simulink model "mosfetbuck_fre"  (R2014a)
settings: Solver=ode23tb  StartTime=0.0  StopTime=0.01  FixedStep=1e-08  RelTol=1e-4
PreLoadFcn:
  | %% Set up model sampling rate
  | Ts = 1e-7;
PostLoadFcn:
  | %% Compute the analytic transfer function for comparison purposes
  | % Load model quiecent operating conditions
  | Vin = str2double(get_param('mosfetbuck_fre/DC','Amplitude'));  % input voltage
  | Dq = str2double(get_param('mosfetbuck_fre/Dq','Value'));       % quiecent duty cycle
  | 
  | % Load model parameters
  | L = str2double(get_param('mosfetbuck_fre/L','Inductance'));    % Henrys
  | C = str2double(get_param('mosfetbuck_fre/C','Capacitance'));   % Farads
  | R = str2double(get_param('mosfetbuck_fre/Load','Resistance')); % Ohms
  | 
  | % Compute transfer function
  | GDnum = 1;
  | GDden = [L*C, L/R,1];
  | GD0 = Vin;
  | 
  | GDbuck = GD0*tf(GDnum,GDden);
InitFcn:
  | %% Set up model sampling rate
  | Ts = 1e-7;
libraries: powerlib x10, powerlib_meascontrol x1
settings Model: Creator=cosorio  LastModifiedBy=cosorio
settings DataIOCC: LimitDataPoints=off  SaveOutput=off  SignalLogging=off  SaveTime=off
settings OptimizationCC: ExpressionDepthLimit=2147483647
settings DebuggingCC: UnderspecifiedInitializationDetection=Classic  SolverPrmCheckMsg=none  FcnCallInpInsideContextMsg=UseLocalSettings  StateNameClashWarn=warning
settings GRTTargetCC: CombineOutputUpdateFcns=off  GRTInterface=on

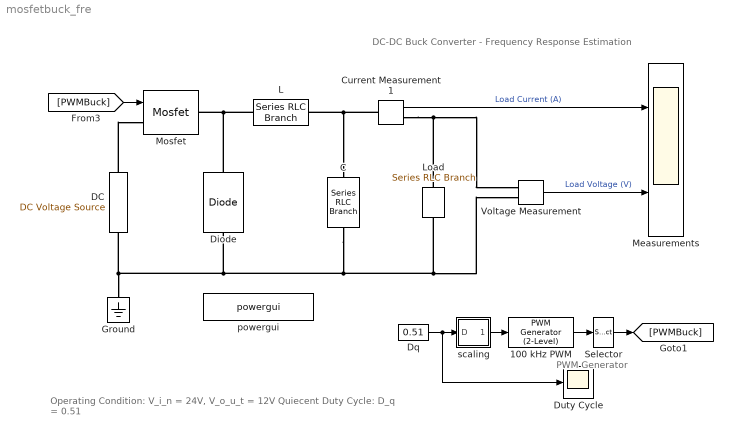
== system mosfetbuck_fre ==
  note: DC-DC Buck Converter - Frequency Response Estimation
  note: Operating Condition: V_i_n = 24V, V_o_u_t = 12V
      | Quiecent Duty Cycle: D_q = 0.51
  note: PWM Generator
  100 kHz PWM : powerlib_meascontrol/Pulse & Signal Generators/PWM Generator (2-Level)  ModulatorType=Single-phase half-bridge (2 pulses)  ModulatorMode=Unsynchronized  nF=27  Fc=1e5  ModulatingSignals=off  m=0.8  Freq=60  Phase=0  Ts=Ts
  C : powerlib/Elements/Series RLC Branch  LConnTagsString=__new0  RConnTagsString=__new0  BranchType=RC  Resistance=0.005  Inductance=30e-6  SetiL0=off  InitialCurrent=0  Capacitance=120e-6  Setx0=off  InitialVoltage=0  Measurements=None
  Current Measurement1 : powerlib/Measurements/Current Measurement  PhasorSimulation=off  OutputType=Complex  PSBequivalent=0
  DC : powerlib/Electrical Sources/DC Voltage Source  Amplitude=24  Measurements=None
  Diode : powerlib/Power Electronics/Diode  Ron=0.01  Lon=0  Vf=0.7  IC=0  UseSnubber=off  Rs=1e5  Cs=250e-9  Measurements=off
  Dq : Constant  Value=0.51  SampleTime=Ts
  Duty Cycle : Scope
      settings: YMin=0  YMax=1  SaveName=DutyCycle  Decimation=10
  Ground : powerlib/Elements/Ground  LConnTagsString=a
  L : powerlib/Elements/Series RLC Branch  LConnTagsString=__new0  RConnTagsString=__new0  BranchType=RL  Resistance=0.001  Inductance=23e-6  SetiL0=off  InitialCurrent=0  Capacitance=1e-6  Setx0=off  InitialVoltage=0  Measurements=None
  Load : powerlib/Elements/Series RLC Branch  LConnTagsString=__new0  RConnTagsString=__new0  BranchType=R  Resistance=1  Inductance=30e-6  SetiL0=off  InitialCurrent=0  Capacitance=100e-6  Setx0=off  InitialVoltage=0  Measurements=None
  Measurements : Scope  NumInputPorts=2
      settings: YMin=0~0  YMax=20~20  Decimation=10
  Mosfet : powerlib/Power Electronics/Mosfet  Ron=0.001  Lon=0  Rd=0.01  Vfd=0.7  IC=0  Rs=1e5  Cs=inf  Measurements=off
  Selector : Selector  InputPortWidth=2  Indices=[1]
  Voltage Measurement : powerlib/Measurements/Voltage Measurement  PhasorSimulation=off  OutputType=Complex  PSBequivalent=0
  powergui : powerlib/powergui  Priority=1  SimulationMode=Discrete  SolverType=Tustin  SampleTime=Ts  frequency=60  SPID=off  DisableSnubberDevices=on  DisableRonSwitches=on  DisableVfSwitches=off  SwTol=0  Interpol=off  DisplayEquations=off  Ts=0  methode=off  frequencyindice=0  Pbase=100e6  ErrMax=1e-4  Iterations=50  UnitsV=kV  UnitsW=MW  FunctionMessages=off  echomessages=off  HookPort=off  EnableUseOfTLC=off  x0status=blocks  RestoreLinks=warning  ResistiveCurrentMeasurement=off  Frange=[0:2:500]  Ylog=off  Xlog=on  ShowGrid=off  save=off  variable=ZData  structure=0  ZoomFFT=on  StartTime=0.0  cycles=1  DisplayStyle=1  fundamental=60  FreqAxis=off  MaxFrequency=1000  frequencyindicesteady=1  RmsSteady=1  display=off
  scaling : Subsystem
  wires:
  Voltage Measurement/1 -> Measurements/2  "Load Voltage (V)"
  100 kHz PWM/1 -> Selector/1
  Dq/1 -> scaling/1(D), Duty Cycle/1
  [PWMBuck] -> Mosfet/1
  Current Measurement1/1 -> Measurements/1  "Load Current (A)"
  Selector/1 -> [PWMBuck]
  scaling/1(m) -> 100 kHz PWM/1
  connections:
  DC/RConn1 -- Mosfet/LConn1
  L/RConn1 -- Mosfet/RConn1 -- Diode/RConn1
  Voltage Measurement/LConn2 -- Load/LConn1 -- C/RConn1 -- Diode/LConn1 -- Ground/LConn1 -- DC/LConn1
  Current Measurement1/RConn1 -- Voltage Measurement/LConn1 -- Load/RConn1
  Current Measurement1/LConn1 -- C/LConn1 -- L/LConn1

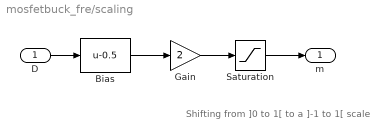
== system mosfetbuck_fre/scaling ==
  note: Shifting from ]0 to 1[ to a ]-1 to 1[ scale
  D : Inport
  Bias : Bias  Bias=-0.5
  Gain : Gain  Gain=2
  Saturation : Saturate  UpperLimit=1  LowerLimit=-1
  m : Outport
  wires:
  Bias/1 -> Gain/1
  D/1 -> Bias/1
  Gain/1 -> Saturation/1
  Saturation/1 -> m/1
